simulink model "compressor_2_stages_test_sim"  (R2017b)
settings: Solver=ode23tb  StartTime=0.0  StopTime=0  MaxStep=0.2  RelTol=1e-3
undefined symbols (not defined in the file or in its folder): BaCl2, gas, liquid, NH3, P, T
libraries: thermochemical x14
settings Model: Creator=ferru  LastModifiedBy=fferrucc
settings SolverCC: AlgebraicLoopSolver=LineSearch

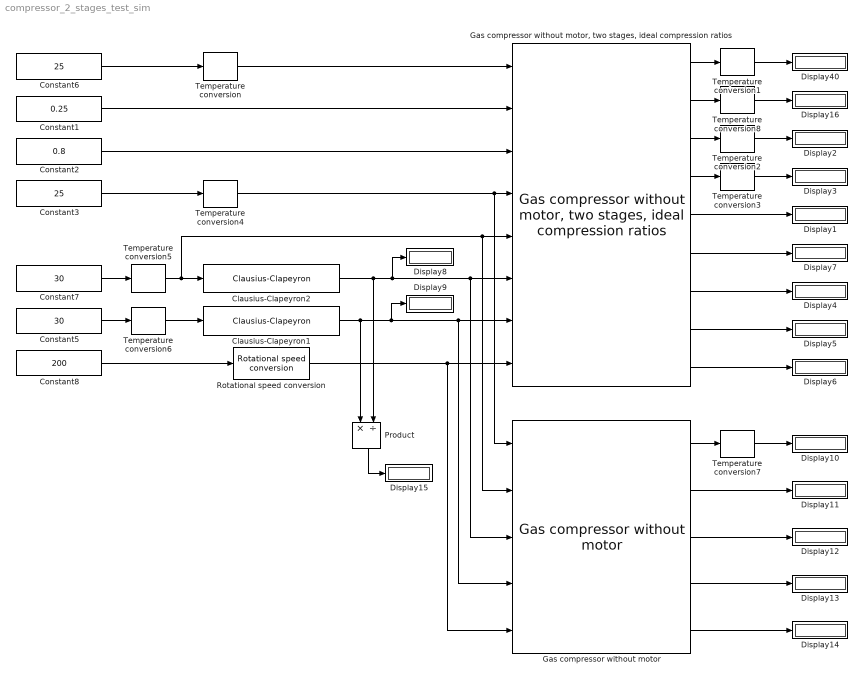
== system compressor_2_stages_test_sim ==
  Clausius-Clapeyron1 : thermochemical/Thermodynamic fluid properties/Clausius-Clapeyron  sel_1=P(T)  sel_2=NH3(liquid)/NH3(gas)
      settings: SourceProductName=@ Thermochemical
  Clausius-Clapeyron2 : thermochemical/Thermodynamic fluid properties/Clausius-Clapeyron  sel_1=P(T)  sel_2=BaCl2/NH3
      settings: SourceProductName=@ Thermochemical
  Constant1 : Constant  Value=0.25
  Constant2 : Constant  Value=0.8
  Constant3 : Constant  Value=25
  Constant5 : Constant  Value=30
  Constant6 : Constant  Value=25
  Constant7 : Constant  Value=30
  Constant8 : Constant  Value=200
  Display{1..16,40} (17 alike) : Display
  Gas compressor without motor : thermochemical/Compression/Gas compressor without motor  fluid=fluid  eta_IS=0.7  CL=0.03  eta_mech=0.9  dVswept_m3_h=6  dVswept_rmp=1500
      settings: SourceProductName=@ Thermochemical
  "Gas compressor without motor, two stages, ideal compression ratios" : thermochemical/Compression/Gas compressor without motor, two stages, ideal compression ratios  fluid=fluid  eta_IS=0.7  CL=0.03  eta_mech=0.9  dVswept_m3_h=6  dVswept_rmp=1500
      settings: SourceProductName=@ Thermochemical
  Product : Product  Inputs=*/
  Rotational speed conversion : thermochemical/Conversions/Rotational speed conversion  sel=rpm --> rad/sec
      settings: SourceProductName=@ Thermochemical
  Temperature conversion{,4..6} (4 alike) : thermochemical/Conversions/Temperature conversion  sel=°C --> K
      settings: SourceProductName=@ Thermochemical
  Temperature conversion{1..3,7..8} (5 alike) : thermochemical/Conversions/Temperature conversion  sel=K --> °C
      settings: SourceProductName=@ Thermochemical
  wires:
  Constant6/1 -> Temperature conversion/1
  Constant1/1 -> "Gas compressor without motor, two stages, ideal compression ratios"/2
  Constant2/1 -> "Gas compressor without motor, two stages, ideal compression ratios"/3
  Constant3/1 -> Temperature conversion4/1
  Constant8/1 -> Rotational speed conversion/1
  "Gas compressor without motor, two stages, ideal compression ratios"/1 -> Temperature conversion1/1
  "Gas compressor without motor, two stages, ideal compression ratios"/5 -> Display1/1
  "Gas compressor without motor, two stages, ideal compression ratios"/3 -> Temperature conversion2/1
  "Gas compressor without motor, two stages, ideal compression ratios"/4 -> Temperature conversion3/1
  "Gas compressor without motor, two stages, ideal compression ratios"/9 -> Display6/1
  "Gas compressor without motor, two stages, ideal compression ratios"/8 -> Display5/1
  "Gas compressor without motor, two stages, ideal compression ratios"/7 -> Display4/1
  "Gas compressor without motor, two stages, ideal compression ratios"/6 -> Display7/1
  Temperature conversion/1 -> "Gas compressor without motor, two stages, ideal compression ratios"/1
  Temperature conversion1/1 -> Display40/1
  Temperature conversion2/1 -> Display2/1
  Temperature conversion3/1 -> Display3/1
  Clausius-Clapeyron2/1 -> Product/2, Display8/1, Gas compressor without motor/3, "Gas compressor without motor, two stages, ideal compression ratios"/6
  Clausius-Clapeyron1/1 -> Display9/1, Gas compressor without motor/4, "Gas compressor without motor, two stages, ideal compression ratios"/7, Product/1
  Constant5/1 -> Temperature conversion6/1
  Constant7/1 -> Temperature conversion5/1
  Rotational speed conversion/1 -> Gas compressor without motor/5, "Gas compressor without motor, two stages, ideal compression ratios"/8
  Temperature conversion4/1 -> Gas compressor without motor/1, "Gas compressor without motor, two stages, ideal compression ratios"/4
  Temperature conversion5/1 -> Gas compressor without motor/2, "Gas compressor without motor, two stages, ideal compression ratios"/5, Clausius-Clapeyron2/1
  Temperature conversion6/1 -> Clausius-Clapeyron1/1
  Gas compressor without motor/1 -> Temperature conversion7/1
  Gas compressor without motor/2 -> Display11/1
  Gas compressor without motor/3 -> Display12/1
  Gas compressor without motor/4 -> Display13/1
  Gas compressor without motor/5 -> Display14/1
  Temperature conversion7/1 -> Display10/1
  Product/1 -> Display15/1
  Temperature conversion8/1 -> Display16/1
  "Gas compressor without motor, two stages, ideal compression ratios"/2 -> Temperature conversion8/1
